simulink model "test_one"  (R2016a)
settings: Solver=ode15s  StartTime=0.0  StopTime=1000  RelTol=1e-3
libraries: simCryogenics_lib x11, nesl_utility x8
settings Model: Creator=FB229602  LastModifiedBy=FB229602
settings DataIOCC: LimitDataPoints=on  SaveFormat=Array
settings HardwareCC: ProdBitPerPointer=32  ProdLargestAtomicFloat=None  ProdIntDivRoundTo=Undefined  ProdEndianess=Unspecified  ProdWordSize=32  ProdHWDeviceType=32-bit Generic
settings ModelReferenceCC: PropagateSignalLabelsOutOfModel=off
settings ConfigComp: CovModelRefEnable=Off
settings SimscapeCC: SimscapeLogType=all

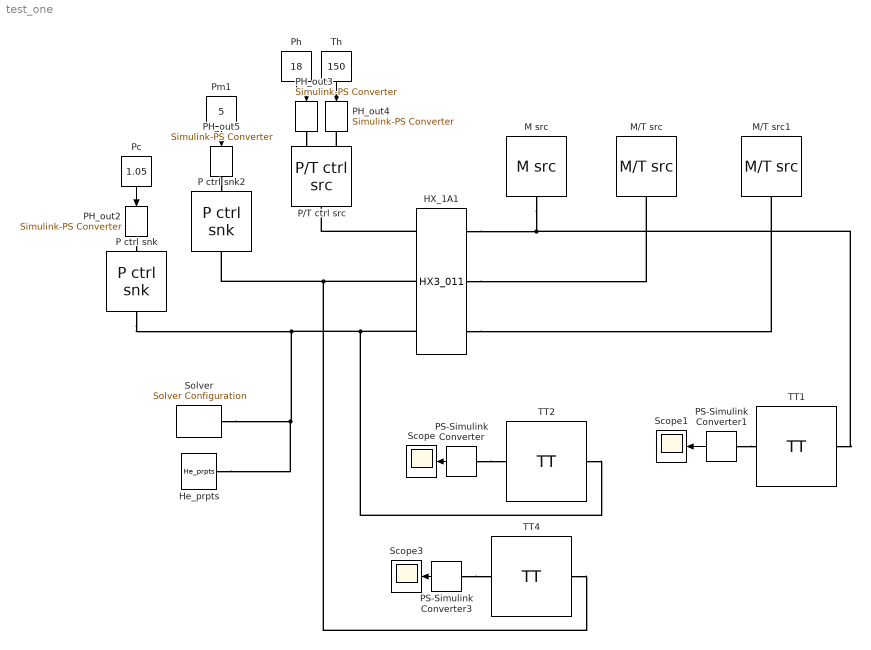
== system test_one ==
  HX_1A1 : simCryogenics_lib/Elements/HX3_011  N=9  Vh=1 m^3  Vm=1 m^3  Vc=1 m^3  M=1000 kg  Kh=0 s*bar/kg  Km=0 s*bar/kg  Kc=0 s*bar/kg  hh_m=1e5 J/s/K  hh_c=1e5 J/s/K  hm_c=1 J/s/K  Th0=150 K  Ph0=18 bar  Mh0=1 kg/s  Tm0=89 K  Pm0=5 bar  Mm0=0.650 kg/s  Tc0=89 K  Pc0=1.05 bar  Mc0=0.650 kg/s  sensh=0  sensm=1  sensc=1
  He_prpts : simCryogenics_lib/Utilities/He_prpts  P_min=0.1 bar  P_max=20 bar  T_min=50 K  T_max=320 K  N=100  Mol=4.0026 * 10 ^ (- 3) kg/mol
  M src : simCryogenics_lib/Sources_Sinks/M src  M=1 kg/s
  M/T src : simCryogenics_lib/Sources_Sinks/M//T src  M=0.650 kg/s  T=89 K
  M/T src1 : simCryogenics_lib/Sources_Sinks/M//T src  M=0.650 kg/s  T=89 K
  P ctrl snk : simCryogenics_lib/Sources_Sinks/P ctrl snk
  P ctrl snk2 : simCryogenics_lib/Sources_Sinks/P ctrl snk
  P/T ctrl src : simCryogenics_lib/Sources_Sinks/P//T ctrl src
  PH_out2 : nesl_utility/Simulink-PS Converter  PhysicalDomain=network_engine_domain  SubClassName=ps_input  LeftPortType=input  RightPortType=output  PseudoPeriodic=off  Frequencies=[]  NoiseDistribution=none  NoiseParameters=[]  Unit=bar  AffineConversion=off  InputFiltering=off  SimscapeFilterOrder=1  InputFilterTimeConstant=0.001  UdotUserProvided=1
  PH_out3 : nesl_utility/Simulink-PS Converter  PhysicalDomain=network_engine_domain  SubClassName=ps_input  LeftPortType=input  RightPortType=output  PseudoPeriodic=off  Frequencies=[]  NoiseDistribution=none  NoiseParameters=[]  Unit=bar  AffineConversion=off  InputFiltering=off  SimscapeFilterOrder=1  InputFilterTimeConstant=0.001  UdotUserProvided=1
  PH_out4 : nesl_utility/Simulink-PS Converter  PhysicalDomain=network_engine_domain  SubClassName=ps_input  LeftPortType=input  RightPortType=output  PseudoPeriodic=off  Frequencies=[]  NoiseDistribution=none  NoiseParameters=[]  Unit=K  AffineConversion=off  InputFiltering=off  SimscapeFilterOrder=1  InputFilterTimeConstant=0.001  UdotUserProvided=1
  PH_out5 : nesl_utility/Simulink-PS Converter  PhysicalDomain=network_engine_domain  SubClassName=ps_input  LeftPortType=input  RightPortType=output  PseudoPeriodic=off  Frequencies=[]  NoiseDistribution=none  NoiseParameters=[]  Unit=bar  AffineConversion=off  InputFiltering=off  SimscapeFilterOrder=1  InputFilterTimeConstant=0.001  UdotUserProvided=1
  PS-Simulink Converter : nesl_utility/PS-Simulink Converter  PhysicalDomain=network_engine_domain  SubClassName=ps_output  LeftPortType=input  RightPortType=output  PseudoPeriodic=off  Frequencies=[]  Unit=1  AffineConversion=off
  PS-Simulink Converter1 : nesl_utility/PS-Simulink Converter  PhysicalDomain=network_engine_domain  SubClassName=ps_output  LeftPortType=input  RightPortType=output  PseudoPeriodic=off  Frequencies=[]  Unit=1  AffineConversion=off
  PS-Simulink Converter3 : nesl_utility/PS-Simulink Converter  PhysicalDomain=network_engine_domain  SubClassName=ps_output  LeftPortType=input  RightPortType=output  PseudoPeriodic=off  Frequencies=[]  Unit=1  AffineConversion=off
  Pc : Constant  Value=1.05
  Ph : Constant  Value=18
  Pm1 : Constant  Value=5
  Scope : Scope
  Scope1 : Scope
  Scope3 : Scope
  Solver : nesl_utility/Solver Configuration  PhysicalDomain=network_engine_domain  SubClassName=solver  LeftPortType=input  RightPortType=generic  Accelerate=off  Tones=[]  Harmonics=[]  SimulateNoise=off  Profile=off  UseLocalSampling=off  EnableSwitchedLinearOptims=on  FrequencyDomain=off  UseCCode=off  RelTol=0.001  AbsTol=1e-06  MinStep=1e-09  ToWorkspace=off  RevertToSquareIcSolve=off  NumHomotopyIterations=100  PhasorMode=off  PhasorModeNumHarmonics=1  OverrideAbsTol=off  DoDC=off  ResidualTolerance=1e-09  UseLocalSolver=off  LocalSolverChoice=NE_BACKWARD_EULER_ADVANCER  LocalSolverSampleTime=0.001  DoFixedCost=off  MaxNonlinIter=3  MaxModeIter=2  LinearAlgebra=Sparse  DelaysMemoryBudget=1024  AutomaticFiltering=on  FilteringTimeConstant=0.001
  TT1 : simCryogenics_lib/Sensors/TT
  TT2 : simCryogenics_lib/Sensors/TT
  TT4 : simCryogenics_lib/Sensors/TT
  Th : Constant  Value=150
  wires:
  Th/1 -> PH_out4/1
  Ph/1 -> PH_out3/1
  Pc/1 -> PH_out2/1
  Pm1/1 -> PH_out5/1
  PS-Simulink Converter/1 -> Scope/1
  PS-Simulink Converter1/1 -> Scope1/1
  PS-Simulink Converter3/1 -> Scope3/1
  connections:
  P ctrl snk/RConn1 -- HX_1A1/LConn1 -- TT2/LConn1 -- He_prpts/RConn1 -- Solver/RConn1
  PH_out5/RConn1 -- P ctrl snk2/LConn1
  P/T ctrl src/LConn2 -- PH_out4/RConn1
  P ctrl snk2/RConn1 -- HX_1A1/LConn2 -- TT4/LConn1
  PH_out2/RConn1 -- P ctrl snk/LConn1
  PH_out3/RConn1 -- P/T ctrl src/LConn1
  HX_1A1/LConn3 -- P/T ctrl src/RConn1
  M src/RConn1 -- HX_1A1/RConn3 -- TT1/LConn1
  HX_1A1/RConn2 -- M/T src/RConn1
  HX_1A1/RConn1 -- M/T src1/RConn1
  PS-Simulink Converter/LConn1 -- TT2/RConn1
  PS-Simulink Converter1/LConn1 -- TT1/RConn1
  PS-Simulink Converter3/LConn1 -- TT4/RConn1
